simulink model "System3"  (R2025a)
settings: Solver=ode113  StartTime=0.0  StopTime=400  FixedStep=0.01  MaxStep=0.1  RelTol=1e-3
libraries: simulink x3784, slpidlib x2
(part 146 of 160)

== system System3/Battery1/Module3/SubModule_1/Cell14/SOCEstimator/SOCEstimator ==
  SOC_Initial : Inport
  Current : Inport  Port=2
  CellCapacity : Inport  Port=3
  Add1 : Sum  Inputs=+-
  Constant : Constant  Value=100  SampleTime=-1
  Constant1 : Constant  Value=3600  SampleTime=-1
  Delay : Delay  DelayLength=1  InitialConditionSource=Input port
      settings: InputPortMap=u0,p4
  Divide : Product  Inputs=*//
  Divide1 : Product  Inputs=*/
  Integrator : Integrator
  Saturation1 : Saturate  UpperLimit=1  LowerLimit=0
  SOC : Outport
  wires:
  Add1/1 -> Saturation1/1
  Constant/1 -> Divide1/2
  Divide1/1 -> Delay/2, Add1/1
  Divide/1 -> Add1/2
  Saturation1/1 -> Delay/1
  SOC_Initial/1 -> Divide1/1
  Current/1 -> Integrator/1
  Delay/1 -> SOC/1
  CellCapacity/1 -> Divide/2
  Constant1/1 -> Divide/3
  Integrator/1 -> Divide/1

== system System3/Battery1/Module3/SubModule_1/Cell15/2RC/RC1 ==
  Current : Inport
  R : Inport  Port=2
  C : Inport  Port=3
  2 : Constant
  Add : Sum
  Divide : Product  Inputs=*/
  Divide1 : Product  Inputs=*/
  Divide2 : Product  Inputs=/*
  Divide3 : Product  Inputs=**
  Integrator1 : Integrator
  Integrator2 : Integrator
  V : Outport
  wires:
  C/1 -> Divide2/1, Divide1/2
  Integrator1/1 -> Divide/1
  Divide1/1 -> Integrator1/1
  Add/1 -> Divide/2
  R/1 -> Add/1, Divide1/1
  Divide2/1 -> Integrator2/1
  Divide/1 -> Divide3/2
  Current/1 -> Divide3/1
  Divide3/1 -> V/1
  Integrator2/1 -> Add/2
  2/1 -> Divide2/2

== system System3/Battery1/Module3/SubModule_1/Cell15/2RC/RC2 ==
  Current : Inport
  R : Inport  Port=2
  C : Inport  Port=3
  2 : Constant
  Add : Sum
  Divide : Product  Inputs=*/
  Divide1 : Product  Inputs=*/
  Divide2 : Product  Inputs=/*
  Divide3 : Product  Inputs=**
  Integrator1 : Integrator
  Integrator2 : Integrator
  V : Outport
  wires:
  2/1 -> Divide2/2
  Integrator2/1 -> Add/2
  Divide3/1 -> V/1
  Current/1 -> Divide3/1
  Divide/1 -> Divide3/2
  Divide2/1 -> Integrator2/1
  R/1 -> Divide1/1, Add/1
  Add/1 -> Divide/2
  Divide1/1 -> Integrator1/1
  Integrator1/1 -> Divide/1
  C/1 -> Divide1/2, Divide2/1

== system System3/Battery1/Module3/SubModule_1/Cell15/2RC/Rint ==
  Current : Inport
  R : Inport  Port=2
  Divide3 : Product  Inputs=**
  V : Outport
  wires:
  R/1 -> Divide3/2
  Current/1 -> Divide3/1
  Divide3/1 -> V/1

== system System3/Battery1/Module3/SubModule_1/Cell15/SOCEstimator/SOCEstimator ==
  SOC_Initial : Inport
  Current : Inport  Port=2
  CellCapacity : Inport  Port=3
  Add1 : Sum  Inputs=+-
  Constant : Constant  Value=100  SampleTime=-1
  Constant1 : Constant  Value=3600  SampleTime=-1
  Delay : Delay  DelayLength=1  InitialConditionSource=Input port
      settings: InputPortMap=u0,p4
  Divide : Product  Inputs=*//
  Divide1 : Product  Inputs=*/
  Integrator : Integrator
  Saturation1 : Saturate  UpperLimit=1  LowerLimit=0
  SOC : Outport
  wires:
  Add1/1 -> Saturation1/1
  Constant/1 -> Divide1/2
  Divide1/1 -> Delay/2, Add1/1
  Divide/1 -> Add1/2
  Saturation1/1 -> Delay/1
  SOC_Initial/1 -> Divide1/1
  Current/1 -> Integrator/1
  Delay/1 -> SOC/1
  CellCapacity/1 -> Divide/2
  Constant1/1 -> Divide/3
  Integrator/1 -> Divide/1

== system System3/Battery1/Module3/SubModule_1/Cell16/2RC/RC1 ==
  Current : Inport
  R : Inport  Port=2
  C : Inport  Port=3
  2 : Constant
  Add : Sum
  Divide : Product  Inputs=*/
  Divide1 : Product  Inputs=*/
  Divide2 : Product  Inputs=/*
  Divide3 : Product  Inputs=**
  Integrator1 : Integrator
  Integrator2 : Integrator
  V : Outport
  wires:
  C/1 -> Divide2/1, Divide1/2
  Integrator1/1 -> Divide/1
  Divide1/1 -> Integrator1/1
  Add/1 -> Divide/2
  R/1 -> Add/1, Divide1/1
  Divide2/1 -> Integrator2/1
  Divide/1 -> Divide3/2
  Current/1 -> Divide3/1
  Divide3/1 -> V/1
  Integrator2/1 -> Add/2
  2/1 -> Divide2/2

== system System3/Battery1/Module3/SubModule_1/Cell16/2RC/RC2 ==
  Current : Inport
  R : Inport  Port=2
  C : Inport  Port=3
  2 : Constant
  Add : Sum
  Divide : Product  Inputs=*/
  Divide1 : Product  Inputs=*/
  Divide2 : Product  Inputs=/*
  Divide3 : Product  Inputs=**
  Integrator1 : Integrator
  Integrator2 : Integrator
  V : Outport
  wires:
  2/1 -> Divide2/2
  Integrator2/1 -> Add/2
  Divide3/1 -> V/1
  Current/1 -> Divide3/1
  Divide/1 -> Divide3/2
  Divide2/1 -> Integrator2/1
  R/1 -> Divide1/1, Add/1
  Add/1 -> Divide/2
  Divide1/1 -> Integrator1/1
  Integrator1/1 -> Divide/1
  C/1 -> Divide1/2, Divide2/1

== system System3/Battery1/Module3/SubModule_1/Cell16/2RC/Rint ==
  Current : Inport
  R : Inport  Port=2
  Divide3 : Product  Inputs=**
  V : Outport
  wires:
  R/1 -> Divide3/2
  Current/1 -> Divide3/1
  Divide3/1 -> V/1

== system System3/Battery1/Module3/SubModule_1/Cell16/SOCEstimator/SOCEstimator ==
  SOC_Initial : Inport
  Current : Inport  Port=2
  CellCapacity : Inport  Port=3
  Add1 : Sum  Inputs=+-
  Constant : Constant  Value=100  SampleTime=-1
  Constant1 : Constant  Value=3600  SampleTime=-1
  Delay : Delay  DelayLength=1  InitialConditionSource=Input port
      settings: InputPortMap=u0,p4
  Divide : Product  Inputs=*//
  Divide1 : Product  Inputs=*/
  Integrator : Integrator
  Saturation1 : Saturate  UpperLimit=1  LowerLimit=0
  SOC : Outport
  wires:
  Add1/1 -> Saturation1/1
  Constant/1 -> Divide1/2
  Divide1/1 -> Delay/2, Add1/1
  Divide/1 -> Add1/2
  Saturation1/1 -> Delay/1
  SOC_Initial/1 -> Divide1/1
  Current/1 -> Integrator/1
  Delay/1 -> SOC/1
  CellCapacity/1 -> Divide/2
  Constant1/1 -> Divide/3
  Integrator/1 -> Divide/1

== system System3/Battery1/Module3/SubModule_1/Cell17/2RC/RC1 ==
  Current : Inport
  R : Inport  Port=2
  C : Inport  Port=3
  2 : Constant
  Add : Sum
  Divide : Product  Inputs=*/
  Divide1 : Product  Inputs=*/
  Divide2 : Product  Inputs=/*
  Divide3 : Product  Inputs=**
  Integrator1 : Integrator
  Integrator2 : Integrator
  V : Outport
  wires:
  2/1 -> Divide2/2
  Integrator2/1 -> Add/2
  Divide3/1 -> V/1
  Current/1 -> Divide3/1
  Divide/1 -> Divide3/2
  Divide2/1 -> Integrator2/1
  R/1 -> Divide1/1, Add/1
  Add/1 -> Divide/2
  Divide1/1 -> Integrator1/1
  Integrator1/1 -> Divide/1
  C/1 -> Divide1/2, Divide2/1

== system System3/Battery1/Module3/SubModule_1/Cell17/2RC/RC2 ==
  Current : Inport
  R : Inport  Port=2
  C : Inport  Port=3
  2 : Constant
  Add : Sum
  Divide : Product  Inputs=*/
  Divide1 : Product  Inputs=*/
  Divide2 : Product  Inputs=/*
  Divide3 : Product  Inputs=**
  Integrator1 : Integrator
  Integrator2 : Integrator
  V : Outport
  wires:
  C/1 -> Divide2/1, Divide1/2
  Integrator1/1 -> Divide/1
  Divide1/1 -> Integrator1/1
  Add/1 -> Divide/2
  R/1 -> Add/1, Divide1/1
  Divide2/1 -> Integrator2/1
  Divide/1 -> Divide3/2
  Current/1 -> Divide3/1
  Divide3/1 -> V/1
  Integrator2/1 -> Add/2
  2/1 -> Divide2/2

== system System3/Battery1/Module3/SubModule_1/Cell17/2RC/Rint ==
  Current : Inport
  R : Inport  Port=2
  Divide3 : Product  Inputs=**
  V : Outport
  wires:
  Divide3/1 -> V/1
  Current/1 -> Divide3/1
  R/1 -> Divide3/2

== system System3/Battery1/Module3/SubModule_1/Cell17/SOCEstimator/SOCEstimator ==
  SOC_Initial : Inport
  Current : Inport  Port=2
  CellCapacity : Inport  Port=3
  Add1 : Sum  Inputs=+-
  Constant : Constant  Value=100  SampleTime=-1
  Constant1 : Constant  Value=3600  SampleTime=-1
  Delay : Delay  DelayLength=1  InitialConditionSource=Input port
      settings: InputPortMap=u0,p4
  Divide : Product  Inputs=*//
  Divide1 : Product  Inputs=*/
  Integrator : Integrator
  Saturation1 : Saturate  UpperLimit=1  LowerLimit=0
  SOC : Outport
  wires:
  Integrator/1 -> Divide/1
  Constant1/1 -> Divide/3
  CellCapacity/1 -> Divide/2
  Delay/1 -> SOC/1
  Current/1 -> Integrator/1
  SOC_Initial/1 -> Divide1/1
  Saturation1/1 -> Delay/1
  Divide/1 -> Add1/2
  Divide1/1 -> Add1/1, Delay/2
  Constant/1 -> Divide1/2
  Add1/1 -> Saturation1/1

== system System3/Battery1/Module3/SubModule_1/Cell18/2RC/RC1 ==
  Current : Inport
  R : Inport  Port=2
  C : Inport  Port=3
  2 : Constant
  Add : Sum
  Divide : Product  Inputs=*/
  Divide1 : Product  Inputs=*/
  Divide2 : Product  Inputs=/*
  Divide3 : Product  Inputs=**
  Integrator1 : Integrator
  Integrator2 : Integrator
  V : Outport
  wires:
  C/1 -> Divide2/1, Divide1/2
  Integrator1/1 -> Divide/1
  Divide1/1 -> Integrator1/1
  Add/1 -> Divide/2
  R/1 -> Add/1, Divide1/1
  Divide2/1 -> Integrator2/1
  Divide/1 -> Divide3/2
  Current/1 -> Divide3/1
  Divide3/1 -> V/1
  Integrator2/1 -> Add/2
  2/1 -> Divide2/2

== system System3/Battery1/Module3/SubModule_1/Cell18/2RC/RC2 ==
  Current : Inport
  R : Inport  Port=2
  C : Inport  Port=3
  2 : Constant
  Add : Sum
  Divide : Product  Inputs=*/
  Divide1 : Product  Inputs=*/
  Divide2 : Product  Inputs=/*
  Divide3 : Product  Inputs=**
  Integrator1 : Integrator
  Integrator2 : Integrator
  V : Outport
  wires:
  2/1 -> Divide2/2
  Integrator2/1 -> Add/2
  Divide3/1 -> V/1
  Current/1 -> Divide3/1
  Divide/1 -> Divide3/2
  Divide2/1 -> Integrator2/1
  R/1 -> Divide1/1, Add/1
  Add/1 -> Divide/2
  Divide1/1 -> Integrator1/1
  Integrator1/1 -> Divide/1
  C/1 -> Divide1/2, Divide2/1

== system System3/Battery1/Module3/SubModule_1/Cell18/2RC/Rint ==
  Current : Inport
  R : Inport  Port=2
  Divide3 : Product  Inputs=**
  V : Outport
  wires:
  R/1 -> Divide3/2
  Current/1 -> Divide3/1
  Divide3/1 -> V/1

== system System3/Battery1/Module3/SubModule_1/Cell18/SOCEstimator/SOCEstimator ==
  SOC_Initial : Inport
  Current : Inport  Port=2
  CellCapacity : Inport  Port=3
  Add1 : Sum  Inputs=+-
  Constant : Constant  Value=100  SampleTime=-1
  Constant1 : Constant  Value=3600  SampleTime=-1
  Delay : Delay  DelayLength=1  InitialConditionSource=Input port
      settings: InputPortMap=u0,p4
  Divide : Product  Inputs=*//
  Divide1 : Product  Inputs=*/
  Integrator : Integrator
  Saturation1 : Saturate  UpperLimit=1  LowerLimit=0
  SOC : Outport
  wires:
  Add1/1 -> Saturation1/1
  Constant/1 -> Divide1/2
  Divide1/1 -> Delay/2, Add1/1
  Divide/1 -> Add1/2
  Saturation1/1 -> Delay/1
  SOC_Initial/1 -> Divide1/1
  Current/1 -> Integrator/1
  Delay/1 -> SOC/1
  CellCapacity/1 -> Divide/2
  Constant1/1 -> Divide/3
  Integrator/1 -> Divide/1

== system System3/Battery1/Module3/SubModule_1/Cell19/2RC/RC1 ==
  Current : Inport
  R : Inport  Port=2
  C : Inport  Port=3
  2 : Constant
  Add : Sum
  Divide : Product  Inputs=*/
  Divide1 : Product  Inputs=*/
  Divide2 : Product  Inputs=/*
  Divide3 : Product  Inputs=**
  Integrator1 : Integrator
  Integrator2 : Integrator
  V : Outport
  wires:
  2/1 -> Divide2/2
  Integrator2/1 -> Add/2
  Divide3/1 -> V/1
  Current/1 -> Divide3/1
  Divide/1 -> Divide3/2
  Divide2/1 -> Integrator2/1
  R/1 -> Divide1/1, Add/1
  Add/1 -> Divide/2
  Divide1/1 -> Integrator1/1
  Integrator1/1 -> Divide/1
  C/1 -> Divide1/2, Divide2/1

== system System3/Battery1/Module3/SubModule_1/Cell19/2RC/RC2 ==
  Current : Inport
  R : Inport  Port=2
  C : Inport  Port=3
  2 : Constant
  Add : Sum
  Divide : Product  Inputs=*/
  Divide1 : Product  Inputs=*/
  Divide2 : Product  Inputs=/*
  Divide3 : Product  Inputs=**
  Integrator1 : Integrator
  Integrator2 : Integrator
  V : Outport
  wires:
  C/1 -> Divide2/1, Divide1/2
  Integrator1/1 -> Divide/1
  Divide1/1 -> Integrator1/1
  Add/1 -> Divide/2
  R/1 -> Add/1, Divide1/1
  Divide2/1 -> Integrator2/1
  Divide/1 -> Divide3/2
  Current/1 -> Divide3/1
  Divide3/1 -> V/1
  Integrator2/1 -> Add/2
  2/1 -> Divide2/2

== system System3/Battery1/Module3/SubModule_1/Cell19/2RC/Rint ==
  Current : Inport
  R : Inport  Port=2
  Divide3 : Product  Inputs=**
  V : Outport
  wires:
  Divide3/1 -> V/1
  Current/1 -> Divide3/1
  R/1 -> Divide3/2

== system System3/Battery1/Module3/SubModule_1/Cell19/SOCEstimator/SOCEstimator ==
  SOC_Initial : Inport
  Current : Inport  Port=2
  CellCapacity : Inport  Port=3
  Add1 : Sum  Inputs=+-
  Constant : Constant  Value=100  SampleTime=-1
  Constant1 : Constant  Value=3600  SampleTime=-1
  Delay : Delay  DelayLength=1  InitialConditionSource=Input port
      settings: InputPortMap=u0,p4
  Divide : Product  Inputs=*//
  Divide1 : Product  Inputs=*/
  Integrator : Integrator
  Saturation1 : Saturate  UpperLimit=1  LowerLimit=0
  SOC : Outport
  wires:
  Integrator/1 -> Divide/1
  Constant1/1 -> Divide/3
  CellCapacity/1 -> Divide/2
  Delay/1 -> SOC/1
  Current/1 -> Integrator/1
  SOC_Initial/1 -> Divide1/1
  Saturation1/1 -> Delay/1
  Divide/1 -> Add1/2
  Divide1/1 -> Add1/1, Delay/2
  Constant/1 -> Divide1/2
  Add1/1 -> Saturation1/1

== system System3/Battery1/Module3/SubModule_1/Cell2/2RC/RC1 ==
  Current : Inport
  R : Inport  Port=2
  C : Inport  Port=3
  2 : Constant
  Add : Sum
  Divide : Product  Inputs=*/
  Divide1 : Product  Inputs=*/
  Divide2 : Product  Inputs=/*
  Divide3 : Product  Inputs=**
  Integrator1 : Integrator
  Integrator2 : Integrator
  V : Outport
  wires:
  C/1 -> Divide2/1, Divide1/2
  Integrator1/1 -> Divide/1
  Divide1/1 -> Integrator1/1
  Add/1 -> Divide/2
  R/1 -> Add/1, Divide1/1
  Divide2/1 -> Integrator2/1
  Divide/1 -> Divide3/2
  Current/1 -> Divide3/1
  Divide3/1 -> V/1
  Integrator2/1 -> Add/2
  2/1 -> Divide2/2

== system System3/Battery1/Module3/SubModule_1/Cell2/2RC/RC2 ==
  Current : Inport
  R : Inport  Port=2
  C : Inport  Port=3
  2 : Constant
  Add : Sum
  Divide : Product  Inputs=*/
  Divide1 : Product  Inputs=*/
  Divide2 : Product  Inputs=/*
  Divide3 : Product  Inputs=**
  Integrator1 : Integrator
  Integrator2 : Integrator
  V : Outport
  wires:
  2/1 -> Divide2/2
  Integrator2/1 -> Add/2
  Divide3/1 -> V/1
  Current/1 -> Divide3/1
  Divide/1 -> Divide3/2
  Divide2/1 -> Integrator2/1
  R/1 -> Divide1/1, Add/1
  Add/1 -> Divide/2
  Divide1/1 -> Integrator1/1
  Integrator1/1 -> Divide/1
  C/1 -> Divide1/2, Divide2/1

== system System3/Battery1/Module3/SubModule_1/Cell2/2RC/Rint ==
  Current : Inport
  R : Inport  Port=2
  Divide3 : Product  Inputs=**
  V : Outport
  wires:
  R/1 -> Divide3/2
  Current/1 -> Divide3/1
  Divide3/1 -> V/1

== system System3/Battery1/Module3/SubModule_1/Cell2/SOCEstimator/SOCEstimator ==
  SOC_Initial : Inport
  Current : Inport  Port=2
  CellCapacity : Inport  Port=3
  Add1 : Sum  Inputs=+-
  Constant : Constant  Value=100  SampleTime=-1
  Constant1 : Constant  Value=3600  SampleTime=-1
  Delay : Delay  DelayLength=1  InitialConditionSource=Input port
      settings: InputPortMap=u0,p4
  Divide : Product  Inputs=*//
  Divide1 : Product  Inputs=*/
  Integrator : Integrator
  Saturation1 : Saturate  UpperLimit=1  LowerLimit=0
  SOC : Outport
  wires:
  Add1/1 -> Saturation1/1
  Constant/1 -> Divide1/2
  Divide1/1 -> Delay/2, Add1/1
  Divide/1 -> Add1/2
  Saturation1/1 -> Delay/1
  SOC_Initial/1 -> Divide1/1
  Current/1 -> Integrator/1
  Delay/1 -> SOC/1
  CellCapacity/1 -> Divide/2
  Constant1/1 -> Divide/3
  Integrator/1 -> Divide/1

== system System3/Battery1/Module3/SubModule_1/Cell20/2RC/RC1 ==
  Current : Inport
  R : Inport  Port=2
  C : Inport  Port=3
  2 : Constant
  Add : Sum
  Divide : Product  Inputs=*/
  Divide1 : Product  Inputs=*/
  Divide2 : Product  Inputs=/*
  Divide3 : Product  Inputs=**
  Integrator1 : Integrator
  Integrator2 : Integrator
  V : Outport
  wires:
  C/1 -> Divide2/1, Divide1/2
  Integrator1/1 -> Divide/1
  Divide1/1 -> Integrator1/1
  Add/1 -> Divide/2
  R/1 -> Add/1, Divide1/1
  Divide2/1 -> Integrator2/1
  Divide/1 -> Divide3/2
  Current/1 -> Divide3/1
  Divide3/1 -> V/1
  Integrator2/1 -> Add/2
  2/1 -> Divide2/2

== system System3/Battery1/Module3/SubModule_1/Cell20/2RC/RC2 ==
  Current : Inport
  R : Inport  Port=2
  C : Inport  Port=3
  2 : Constant
  Add : Sum
  Divide : Product  Inputs=*/
  Divide1 : Product  Inputs=*/
  Divide2 : Product  Inputs=/*
  Divide3 : Product  Inputs=**
  Integrator1 : Integrator
  Integrator2 : Integrator
  V : Outport
  wires:
  2/1 -> Divide2/2
  Integrator2/1 -> Add/2
  Divide3/1 -> V/1
  Current/1 -> Divide3/1
  Divide/1 -> Divide3/2
  Divide2/1 -> Integrator2/1
  R/1 -> Divide1/1, Add/1
  Add/1 -> Divide/2
  Divide1/1 -> Integrator1/1
  Integrator1/1 -> Divide/1
  C/1 -> Divide1/2, Divide2/1

== system System3/Battery1/Module3/SubModule_1/Cell20/2RC/Rint ==
  Current : Inport
  R : Inport  Port=2
  Divide3 : Product  Inputs=**
  V : Outport
  wires:
  R/1 -> Divide3/2
  Current/1 -> Divide3/1
  Divide3/1 -> V/1

== system System3/Battery1/Module3/SubModule_1/Cell20/SOCEstimator/SOCEstimator ==
  SOC_Initial : Inport
  Current : Inport  Port=2
  CellCapacity : Inport  Port=3
  Add1 : Sum  Inputs=+-
  Constant : Constant  Value=100  SampleTime=-1
  Constant1 : Constant  Value=3600  SampleTime=-1
  Delay : Delay  DelayLength=1  InitialConditionSource=Input port
      settings: InputPortMap=u0,p4
  Divide : Product  Inputs=*//
  Divide1 : Product  Inputs=*/
  Integrator : Integrator
  Saturation1 : Saturate  UpperLimit=1  LowerLimit=0
  SOC : Outport
  wires:
  Add1/1 -> Saturation1/1
  Constant/1 -> Divide1/2
  Divide1/1 -> Delay/2, Add1/1
  Divide/1 -> Add1/2
  Saturation1/1 -> Delay/1
  SOC_Initial/1 -> Divide1/1
  Current/1 -> Integrator/1
  Delay/1 -> SOC/1
  CellCapacity/1 -> Divide/2
  Constant1/1 -> Divide/3
  Integrator/1 -> Divide/1

== system System3/Battery1/Module3/SubModule_1/Cell21/2RC/RC1 ==
  Current : Inport
  R : Inport  Port=2
  C : Inport  Port=3
  2 : Constant
  Add : Sum
  Divide : Product  Inputs=*/
  Divide1 : Product  Inputs=*/
  Divide2 : Product  Inputs=/*
  Divide3 : Product  Inputs=**
  Integrator1 : Integrator
  Integrator2 : Integrator
  V : Outport
  wires:
  2/1 -> Divide2/2
  Integrator2/1 -> Add/2
  Divide3/1 -> V/1
  Current/1 -> Divide3/1
  Divide/1 -> Divide3/2
  Divide2/1 -> Integrator2/1
  R/1 -> Divide1/1, Add/1
  Add/1 -> Divide/2
  Divide1/1 -> Integrator1/1
  Integrator1/1 -> Divide/1
  C/1 -> Divide1/2, Divide2/1

== system System3/Battery1/Module3/SubModule_1/Cell21/2RC/RC2 ==
  Current : Inport
  R : Inport  Port=2
  C : Inport  Port=3
  2 : Constant
  Add : Sum
  Divide : Product  Inputs=*/
  Divide1 : Product  Inputs=*/
  Divide2 : Product  Inputs=/*
  Divide3 : Product  Inputs=**
  Integrator1 : Integrator
  Integrator2 : Integrator
  V : Outport
  wires:
  C/1 -> Divide2/1, Divide1/2
  Integrator1/1 -> Divide/1
  Divide1/1 -> Integrator1/1
  Add/1 -> Divide/2
  R/1 -> Add/1, Divide1/1
  Divide2/1 -> Integrator2/1
  Divide/1 -> Divide3/2
  Current/1 -> Divide3/1
  Divide3/1 -> V/1
  Integrator2/1 -> Add/2
  2/1 -> Divide2/2

== system System3/Battery1/Module3/SubModule_1/Cell21/2RC/Rint ==
  Current : Inport
  R : Inport  Port=2
  Divide3 : Product  Inputs=**
  V : Outport
  wires:
  Divide3/1 -> V/1
  Current/1 -> Divide3/1
  R/1 -> Divide3/2

== system System3/Battery1/Module3/SubModule_1/Cell21/SOCEstimator/SOCEstimator ==
  SOC_Initial : Inport
  Current : Inport  Port=2
  CellCapacity : Inport  Port=3
  Add1 : Sum  Inputs=+-
  Constant : Constant  Value=100  SampleTime=-1
  Constant1 : Constant  Value=3600  SampleTime=-1
  Delay : Delay  DelayLength=1  InitialConditionSource=Input port
      settings: InputPortMap=u0,p4
  Divide : Product  Inputs=*//
  Divide1 : Product  Inputs=*/
  Integrator : Integrator
  Saturation1 : Saturate  UpperLimit=1  LowerLimit=0
  SOC : Outport
  wires:
  Integrator/1 -> Divide/1
  Constant1/1 -> Divide/3
  CellCapacity/1 -> Divide/2
  Delay/1 -> SOC/1
  Current/1 -> Integrator/1
  SOC_Initial/1 -> Divide1/1
  Saturation1/1 -> Delay/1
  Divide/1 -> Add1/2
  Divide1/1 -> Add1/1, Delay/2
  Constant/1 -> Divide1/2
  Add1/1 -> Saturation1/1

== system System3/Battery1/Module3/SubModule_1/Cell22/2RC/RC1 ==
  Current : Inport
  R : Inport  Port=2
  C : Inport  Port=3
  2 : Constant
  Add : Sum
  Divide : Product  Inputs=*/
  Divide1 : Product  Inputs=*/
  Divide2 : Product  Inputs=/*
  Divide3 : Product  Inputs=**
  Integrator1 : Integrator
  Integrator2 : Integrator
  V : Outport
  wires:
  2/1 -> Divide2/2
  Integrator2/1 -> Add/2
  Divide3/1 -> V/1
  Current/1 -> Divide3/1
  Divide/1 -> Divide3/2
  Divide2/1 -> Integrator2/1
  R/1 -> Divide1/1, Add/1
  Add/1 -> Divide/2
  Divide1/1 -> Integrator1/1
  Integrator1/1 -> Divide/1
  C/1 -> Divide1/2, Divide2/1

== system System3/Battery1/Module3/SubModule_1/Cell22/2RC/RC2 ==
  Current : Inport
  R : Inport  Port=2
  C : Inport  Port=3
  2 : Constant
  Add : Sum
  Divide : Product  Inputs=*/
  Divide1 : Product  Inputs=*/
  Divide2 : Product  Inputs=/*
  Divide3 : Product  Inputs=**
  Integrator1 : Integrator
  Integrator2 : Integrator
  V : Outport
  wires:
  C/1 -> Divide2/1, Divide1/2
  Integrator1/1 -> Divide/1
  Divide1/1 -> Integrator1/1
  Add/1 -> Divide/2
  R/1 -> Add/1, Divide1/1
  Divide2/1 -> Integrator2/1
  Divide/1 -> Divide3/2
  Current/1 -> Divide3/1
  Divide3/1 -> V/1
  Integrator2/1 -> Add/2
  2/1 -> Divide2/2

== system System3/Battery1/Module3/SubModule_1/Cell22/2RC/Rint ==
  Current : Inport
  R : Inport  Port=2
  Divide3 : Product  Inputs=**
  V : Outport
  wires:
  Divide3/1 -> V/1
  Current/1 -> Divide3/1
  R/1 -> Divide3/2

== system System3/Battery1/Module3/SubModule_1/Cell22/SOCEstimator/SOCEstimator ==
  SOC_Initial : Inport
  Current : Inport  Port=2
  CellCapacity : Inport  Port=3
  Add1 : Sum  Inputs=+-
  Constant : Constant  Value=100  SampleTime=-1
  Constant1 : Constant  Value=3600  SampleTime=-1
  Delay : Delay  DelayLength=1  InitialConditionSource=Input port
      settings: InputPortMap=u0,p4
  Divide : Product  Inputs=*//
  Divide1 : Product  Inputs=*/
  Integrator : Integrator
  Saturation1 : Saturate  UpperLimit=1  LowerLimit=0
  SOC : Outport
  wires:
  Integrator/1 -> Divide/1
  Constant1/1 -> Divide/3
  CellCapacity/1 -> Divide/2
  Delay/1 -> SOC/1
  Current/1 -> Integrator/1
  SOC_Initial/1 -> Divide1/1
  Saturation1/1 -> Delay/1
  Divide/1 -> Add1/2
  Divide1/1 -> Add1/1, Delay/2
  Constant/1 -> Divide1/2
  Add1/1 -> Saturation1/1

== system System3/Battery1/Module3/SubModule_1/Cell3/2RC/RC1 ==
  Current : Inport
  R : Inport  Port=2
  C : Inport  Port=3
  2 : Constant
  Add : Sum
  Divide : Product  Inputs=*/
  Divide1 : Product  Inputs=*/
  Divide2 : Product  Inputs=/*
  Divide3 : Product  Inputs=**
  Integrator1 : Integrator
  Integrator2 : Integrator
  V : Outport
  wires:
  2/1 -> Divide2/2
  Integrator2/1 -> Add/2
  Divide3/1 -> V/1
  Current/1 -> Divide3/1
  Divide/1 -> Divide3/2
  Divide2/1 -> Integrator2/1
  R/1 -> Divide1/1, Add/1
  Add/1 -> Divide/2
  Divide1/1 -> Integrator1/1
  Integrator1/1 -> Divide/1
  C/1 -> Divide1/2, Divide2/1

== system System3/Battery1/Module3/SubModule_1/Cell3/2RC/RC2 ==
  Current : Inport
  R : Inport  Port=2
  C : Inport  Port=3
  2 : Constant
  Add : Sum
  Divide : Product  Inputs=*/
  Divide1 : Product  Inputs=*/
  Divide2 : Product  Inputs=/*
  Divide3 : Product  Inputs=**
  Integrator1 : Integrator
  Integrator2 : Integrator
  V : Outport
  wires:
  C/1 -> Divide2/1, Divide1/2
  Integrator1/1 -> Divide/1
  Divide1/1 -> Integrator1/1
  Add/1 -> Divide/2
  R/1 -> Add/1, Divide1/1
  Divide2/1 -> Integrator2/1
  Divide/1 -> Divide3/2
  Current/1 -> Divide3/1
  Divide3/1 -> V/1
  Integrator2/1 -> Add/2
  2/1 -> Divide2/2

== system System3/Battery1/Module3/SubModule_1/Cell3/2RC/Rint ==
  Current : Inport
  R : Inport  Port=2
  Divide3 : Product  Inputs=**
  V : Outport
  wires:
  Divide3/1 -> V/1
  Current/1 -> Divide3/1
  R/1 -> Divide3/2

== system System3/Battery1/Module3/SubModule_1/Cell3/SOCEstimator/SOCEstimator ==
  SOC_Initial : Inport
  Current : Inport  Port=2
  CellCapacity : Inport  Port=3
  Add1 : Sum  Inputs=+-
  Constant : Constant  Value=100  SampleTime=-1
  Constant1 : Constant  Value=3600  SampleTime=-1
  Delay : Delay  DelayLength=1  InitialConditionSource=Input port
      settings: InputPortMap=u0,p4
  Divide : Product  Inputs=*//
  Divide1 : Product  Inputs=*/
  Integrator : Integrator
  Saturation1 : Saturate  UpperLimit=1  LowerLimit=0
  SOC : Outport
  wires:
  Integrator/1 -> Divide/1
  Constant1/1 -> Divide/3
  CellCapacity/1 -> Divide/2
  Delay/1 -> SOC/1
  Current/1 -> Integrator/1
  SOC_Initial/1 -> Divide1/1
  Saturation1/1 -> Delay/1
  Divide/1 -> Add1/2
  Divide1/1 -> Add1/1, Delay/2
  Constant/1 -> Divide1/2
  Add1/1 -> Saturation1/1

== system System3/Battery1/Module3/SubModule_1/Cell4/2RC/RC1 ==
  Current : Inport
  R : Inport  Port=2
  C : Inport  Port=3
  2 : Constant
  Add : Sum
  Divide : Product  Inputs=*/
  Divide1 : Product  Inputs=*/
  Divide2 : Product  Inputs=/*
  Divide3 : Product  Inputs=**
  Integrator1 : Integrator
  Integrator2 : Integrator
  V : Outport
  wires:
  C/1 -> Divide2/1, Divide1/2
  Integrator1/1 -> Divide/1
  Divide1/1 -> Integrator1/1
  Add/1 -> Divide/2
  R/1 -> Add/1, Divide1/1
  Divide2/1 -> Integrator2/1
  Divide/1 -> Divide3/2
  Current/1 -> Divide3/1
  Divide3/1 -> V/1
  Integrator2/1 -> Add/2
  2/1 -> Divide2/2

== system System3/Battery1/Module3/SubModule_1/Cell4/2RC/RC2 ==
  Current : Inport
  R : Inport  Port=2
  C : Inport  Port=3
  2 : Constant
  Add : Sum
  Divide : Product  Inputs=*/
  Divide1 : Product  Inputs=*/
  Divide2 : Product  Inputs=/*
  Divide3 : Product  Inputs=**
  Integrator1 : Integrator
  Integrator2 : Integrator
  V : Outport
  wires:
  2/1 -> Divide2/2
  Integrator2/1 -> Add/2
  Divide3/1 -> V/1
  Current/1 -> Divide3/1
  Divide/1 -> Divide3/2
  Divide2/1 -> Integrator2/1
  R/1 -> Divide1/1, Add/1
  Add/1 -> Divide/2
  Divide1/1 -> Integrator1/1
  Integrator1/1 -> Divide/1
  C/1 -> Divide1/2, Divide2/1

== system System3/Battery1/Module3/SubModule_1/Cell4/2RC/Rint ==
  Current : Inport
  R : Inport  Port=2
  Divide3 : Product  Inputs=**
  V : Outport
  wires:
  R/1 -> Divide3/2
  Current/1 -> Divide3/1
  Divide3/1 -> V/1

== system System3/Battery1/Module3/SubModule_1/Cell4/SOCEstimator/SOCEstimator ==
  SOC_Initial : Inport
  Current : Inport  Port=2
  CellCapacity : Inport  Port=3
  Add1 : Sum  Inputs=+-
  Constant : Constant  Value=100  SampleTime=-1
  Constant1 : Constant  Value=3600  SampleTime=-1
  Delay : Delay  DelayLength=1  InitialConditionSource=Input port
      settings: InputPortMap=u0,p4
  Divide : Product  Inputs=*//
  Divide1 : Product  Inputs=*/
  Integrator : Integrator
  Saturation1 : Saturate  UpperLimit=1  LowerLimit=0
  SOC : Outport
  wires:
  Add1/1 -> Saturation1/1
  Constant/1 -> Divide1/2
  Divide1/1 -> Delay/2, Add1/1
  Divide/1 -> Add1/2
  Saturation1/1 -> Delay/1
  SOC_Initial/1 -> Divide1/1
  Current/1 -> Integrator/1
  Delay/1 -> SOC/1
  CellCapacity/1 -> Divide/2
  Constant1/1 -> Divide/3
  Integrator/1 -> Divide/1

== system System3/Battery1/Module3/SubModule_1/Cell5/2RC/RC1 ==
  Current : Inport
  R : Inport  Port=2
  C : Inport  Port=3
  2 : Constant
  Add : Sum
  Divide : Product  Inputs=*/
  Divide1 : Product  Inputs=*/
  Divide2 : Product  Inputs=/*
  Divide3 : Product  Inputs=**
  Integrator1 : Integrator
  Integrator2 : Integrator
  V : Outport
  wires:
  2/1 -> Divide2/2
  Integrator2/1 -> Add/2
  Divide3/1 -> V/1
  Current/1 -> Divide3/1
  Divide/1 -> Divide3/2
  Divide2/1 -> Integrator2/1
  R/1 -> Divide1/1, Add/1
  Add/1 -> Divide/2
  Divide1/1 -> Integrator1/1
  Integrator1/1 -> Divide/1
  C/1 -> Divide1/2, Divide2/1

== system System3/Battery1/Module3/SubModule_1/Cell5/2RC/RC2 ==
  Current : Inport
  R : Inport  Port=2
  C : Inport  Port=3
  2 : Constant
  Add : Sum
  Divide : Product  Inputs=*/
  Divide1 : Product  Inputs=*/
  Divide2 : Product  Inputs=/*
  Divide3 : Product  Inputs=**
  Integrator1 : Integrator
  Integrator2 : Integrator
  V : Outport
  wires:
  C/1 -> Divide2/1, Divide1/2
  Integrator1/1 -> Divide/1
  Divide1/1 -> Integrator1/1
  Add/1 -> Divide/2
  R/1 -> Add/1, Divide1/1
  Divide2/1 -> Integrator2/1
  Divide/1 -> Divide3/2
  Current/1 -> Divide3/1
  Divide3/1 -> V/1
  Integrator2/1 -> Add/2
  2/1 -> Divide2/2

== system System3/Battery1/Module3/SubModule_1/Cell5/2RC/Rint ==
  Current : Inport
  R : Inport  Port=2
  Divide3 : Product  Inputs=**
  V : Outport
  wires:
  Divide3/1 -> V/1
  Current/1 -> Divide3/1
  R/1 -> Divide3/2

== system System3/Battery1/Module3/SubModule_1/Cell5/SOCEstimator/SOCEstimator ==
  SOC_Initial : Inport
  Current : Inport  Port=2
  CellCapacity : Inport  Port=3
  Add1 : Sum  Inputs=+-
  Constant : Constant  Value=100  SampleTime=-1
  Constant1 : Constant  Value=3600  SampleTime=-1
  Delay : Delay  DelayLength=1  InitialConditionSource=Input port
      settings: InputPortMap=u0,p4
  Divide : Product  Inputs=*//
  Divide1 : Product  Inputs=*/
  Integrator : Integrator
  Saturation1 : Saturate  UpperLimit=1  LowerLimit=0
  SOC : Outport
  wires:
  Integrator/1 -> Divide/1
  Constant1/1 -> Divide/3
  CellCapacity/1 -> Divide/2
  Delay/1 -> SOC/1
  Current/1 -> Integrator/1
  SOC_Initial/1 -> Divide1/1
  Saturation1/1 -> Delay/1
  Divide/1 -> Add1/2
  Divide1/1 -> Add1/1, Delay/2
  Constant/1 -> Divide1/2
  Add1/1 -> Saturation1/1

== system System3/Battery1/Module3/SubModule_1/Cell6/2RC/RC1 ==
  Current : Inport
  R : Inport  Port=2
  C : Inport  Port=3
  2 : Constant
  Add : Sum
  Divide : Product  Inputs=*/
  Divide1 : Product  Inputs=*/
  Divide2 : Product  Inputs=/*
  Divide3 : Product  Inputs=**
  Integrator1 : Integrator
  Integrator2 : Integrator
  V : Outport
  wires:
  C/1 -> Divide2/1, Divide1/2
  Integrator1/1 -> Divide/1
  Divide1/1 -> Integrator1/1
  Add/1 -> Divide/2
  R/1 -> Add/1, Divide1/1
  Divide2/1 -> Integrator2/1
  Divide/1 -> Divide3/2
  Current/1 -> Divide3/1
  Divide3/1 -> V/1
  Integrator2/1 -> Add/2
  2/1 -> Divide2/2

== system System3/Battery1/Module3/SubModule_1/Cell6/2RC/RC2 ==
  Current : Inport
  R : Inport  Port=2
  C : Inport  Port=3
  2 : Constant
  Add : Sum
  Divide : Product  Inputs=*/
  Divide1 : Product  Inputs=*/
  Divide2 : Product  Inputs=/*
  Divide3 : Product  Inputs=**
  Integrator1 : Integrator
  Integrator2 : Integrator
  V : Outport
  wires:
  2/1 -> Divide2/2
  Integrator2/1 -> Add/2
  Divide3/1 -> V/1
  Current/1 -> Divide3/1
  Divide/1 -> Divide3/2
  Divide2/1 -> Integrator2/1
  R/1 -> Divide1/1, Add/1
  Add/1 -> Divide/2
  Divide1/1 -> Integrator1/1
  Integrator1/1 -> Divide/1
  C/1 -> Divide1/2, Divide2/1

== system System3/Battery1/Module3/SubModule_1/Cell6/2RC/Rint ==
  Current : Inport
  R : Inport  Port=2
  Divide3 : Product  Inputs=**
  V : Outport
  wires:
  R/1 -> Divide3/2
  Current/1 -> Divide3/1
  Divide3/1 -> V/1

== system System3/Battery1/Module3/SubModule_1/Cell6/SOCEstimator/SOCEstimator ==
  SOC_Initial : Inport
  Current : Inport  Port=2
  CellCapacity : Inport  Port=3
  Add1 : Sum  Inputs=+-
  Constant : Constant  Value=100  SampleTime=-1
  Constant1 : Constant  Value=3600  SampleTime=-1
  Delay : Delay  DelayLength=1  InitialConditionSource=Input port
      settings: InputPortMap=u0,p4
  Divide : Product  Inputs=*//
  Divide1 : Product  Inputs=*/
  Integrator : Integrator
  Saturation1 : Saturate  UpperLimit=1  LowerLimit=0
  SOC : Outport
  wires:
  Add1/1 -> Saturation1/1
  Constant/1 -> Divide1/2
  Divide1/1 -> Delay/2, Add1/1
  Divide/1 -> Add1/2
  Saturation1/1 -> Delay/1
  SOC_Initial/1 -> Divide1/1
  Current/1 -> Integrator/1
  Delay/1 -> SOC/1
  CellCapacity/1 -> Divide/2
  Constant1/1 -> Divide/3
  Integrator/1 -> Divide/1

== system System3/Battery1/Module3/SubModule_1/Cell7/2RC/RC1 ==
  Current : Inport
  R : Inport  Port=2
  C : Inport  Port=3
  2 : Constant
  Add : Sum
  Divide : Product  Inputs=*/
  Divide1 : Product  Inputs=*/
  Divide2 : Product  Inputs=/*
  Divide3 : Product  Inputs=**
  Integrator1 : Integrator
  Integrator2 : Integrator
  V : Outport
  wires:
  C/1 -> Divide2/1, Divide1/2
  Integrator1/1 -> Divide/1
  Divide1/1 -> Integrator1/1
  Add/1 -> Divide/2
  R/1 -> Add/1, Divide1/1
  Divide2/1 -> Integrator2/1
  Divide/1 -> Divide3/2
  Current/1 -> Divide3/1
  Divide3/1 -> V/1
  Integrator2/1 -> Add/2
  2/1 -> Divide2/2

== system System3/Battery1/Module3/SubModule_1/Cell7/2RC/RC2 ==
  Current : Inport
  R : Inport  Port=2
  C : Inport  Port=3
  2 : Constant
  Add : Sum
  Divide : Product  Inputs=*/
  Divide1 : Product  Inputs=*/
  Divide2 : Product  Inputs=/*
  Divide3 : Product  Inputs=**
  Integrator1 : Integrator
  Integrator2 : Integrator
  V : Outport
  wires:
  2/1 -> Divide2/2
  Integrator2/1 -> Add/2
  Divide3/1 -> V/1
  Current/1 -> Divide3/1
  Divide/1 -> Divide3/2
  Divide2/1 -> Integrator2/1
  R/1 -> Divide1/1, Add/1
  Add/1 -> Divide/2
  Divide1/1 -> Integrator1/1
  Integrator1/1 -> Divide/1
  C/1 -> Divide1/2, Divide2/1

== system System3/Battery1/Module3/SubModule_1/Cell7/2RC/Rint ==
  Current : Inport
  R : Inport  Port=2
  Divide3 : Product  Inputs=**
  V : Outport
  wires:
  R/1 -> Divide3/2
  Current/1 -> Divide3/1
  Divide3/1 -> V/1

== system System3/Battery1/Module3/SubModule_1/Cell7/SOCEstimator/SOCEstimator ==
  SOC_Initial : Inport
  Current : Inport  Port=2
  CellCapacity : Inport  Port=3
  Add1 : Sum  Inputs=+-
  Constant : Constant  Value=100  SampleTime=-1
  Constant1 : Constant  Value=3600  SampleTime=-1
  Delay : Delay  DelayLength=1  InitialConditionSource=Input port
      settings: InputPortMap=u0,p4
  Divide : Product  Inputs=*//
  Divide1 : Product  Inputs=*/
  Integrator : Integrator
  Saturation1 : Saturate  UpperLimit=1  LowerLimit=0
  SOC : Outport
  wires:
  Add1/1 -> Saturation1/1
  Constant/1 -> Divide1/2
  Divide1/1 -> Delay/2, Add1/1
  Divide/1 -> Add1/2
  Saturation1/1 -> Delay/1
  SOC_Initial/1 -> Divide1/1
  Current/1 -> Integrator/1
  Delay/1 -> SOC/1
  CellCapacity/1 -> Divide/2
  Constant1/1 -> Divide/3
  Integrator/1 -> Divide/1

== system System3/Battery1/Module3/SubModule_1/Cell8/2RC/RC1 ==
  Current : Inport
  R : Inport  Port=2
  C : Inport  Port=3
  2 : Constant
  Add : Sum
  Divide : Product  Inputs=*/
  Divide1 : Product  Inputs=*/
  Divide2 : Product  Inputs=/*
  Divide3 : Product  Inputs=**
  Integrator1 : Integrator
  Integrator2 : Integrator
  V : Outport
  wires:
  2/1 -> Divide2/2
  Integrator2/1 -> Add/2
  Divide3/1 -> V/1
  Current/1 -> Divide3/1
  Divide/1 -> Divide3/2
  Divide2/1 -> Integrator2/1
  R/1 -> Divide1/1, Add/1
  Add/1 -> Divide/2
  Divide1/1 -> Integrator1/1
  Integrator1/1 -> Divide/1
  C/1 -> Divide1/2, Divide2/1

== system System3/Battery1/Module3/SubModule_1/Cell8/2RC/RC2 ==
  Current : Inport
  R : Inport  Port=2
  C : Inport  Port=3
  2 : Constant
  Add : Sum
  Divide : Product  Inputs=*/
  Divide1 : Product  Inputs=*/
  Divide2 : Product  Inputs=/*
  Divide3 : Product  Inputs=**
  Integrator1 : Integrator
  Integrator2 : Integrator
  V : Outport
  wires:
  C/1 -> Divide2/1, Divide1/2
  Integrator1/1 -> Divide/1
  Divide1/1 -> Integrator1/1
  Add/1 -> Divide/2
  R/1 -> Add/1, Divide1/1
  Divide2/1 -> Integrator2/1
  Divide/1 -> Divide3/2
  Current/1 -> Divide3/1
  Divide3/1 -> V/1
  Integrator2/1 -> Add/2
  2/1 -> Divide2/2

== system System3/Battery1/Module3/SubModule_1/Cell8/2RC/Rint ==
  Current : Inport
  R : Inport  Port=2
  Divide3 : Product  Inputs=**
  V : Outport
  wires:
  Divide3/1 -> V/1
  Current/1 -> Divide3/1
  R/1 -> Divide3/2

== system System3/Battery1/Module3/SubModule_1/Cell8/SOCEstimator/SOCEstimator ==
  SOC_Initial : Inport
  Current : Inport  Port=2
  CellCapacity : Inport  Port=3
  Add1 : Sum  Inputs=+-
  Constant : Constant  Value=100  SampleTime=-1
  Constant1 : Constant  Value=3600  SampleTime=-1
  Delay : Delay  DelayLength=1  InitialConditionSource=Input port
      settings: InputPortMap=u0,p4
  Divide : Product  Inputs=*//
  Divide1 : Product  Inputs=*/
  Integrator : Integrator
  Saturation1 : Saturate  UpperLimit=1  LowerLimit=0
  SOC : Outport
  wires:
  Integrator/1 -> Divide/1
  Constant1/1 -> Divide/3
  CellCapacity/1 -> Divide/2
  Delay/1 -> SOC/1
  Current/1 -> Integrator/1
  SOC_Initial/1 -> Divide1/1
  Saturation1/1 -> Delay/1
  Divide/1 -> Add1/2
  Divide1/1 -> Add1/1, Delay/2
  Constant/1 -> Divide1/2
  Add1/1 -> Saturation1/1

== system System3/Battery1/Module3/SubModule_1/Cell9/2RC/RC1 ==
  Current : Inport
  R : Inport  Port=2
  C : Inport  Port=3
  2 : Constant
  Add : Sum
  Divide : Product  Inputs=*/
  Divide1 : Product  Inputs=*/
  Divide2 : Product  Inputs=/*
  Divide3 : Product  Inputs=**
  Integrator1 : Integrator
  Integrator2 : Integrator
  V : Outport
  wires:
  C/1 -> Divide2/1, Divide1/2
  Integrator1/1 -> Divide/1
  Divide1/1 -> Integrator1/1
  Add/1 -> Divide/2
  R/1 -> Add/1, Divide1/1
  Divide2/1 -> Integrator2/1
  Divide/1 -> Divide3/2
  Current/1 -> Divide3/1
  Divide3/1 -> V/1
  Integrator2/1 -> Add/2
  2/1 -> Divide2/2

== system System3/Battery1/Module3/SubModule_1/Cell9/2RC/RC2 ==
  Current : Inport
  R : Inport  Port=2
  C : Inport  Port=3
  2 : Constant
  Add : Sum
  Divide : Product  Inputs=*/
  Divide1 : Product  Inputs=*/
  Divide2 : Product  Inputs=/*
  Divide3 : Product  Inputs=**
  Integrator1 : Integrator
  Integrator2 : Integrator
  V : Outport
  wires:
  2/1 -> Divide2/2
  Integrator2/1 -> Add/2
  Divide3/1 -> V/1
  Current/1 -> Divide3/1
  Divide/1 -> Divide3/2
  Divide2/1 -> Integrator2/1
  R/1 -> Divide1/1, Add/1
  Add/1 -> Divide/2
  Divide1/1 -> Integrator1/1
  Integrator1/1 -> Divide/1
  C/1 -> Divide1/2, Divide2/1

== system System3/Battery1/Module3/SubModule_1/Cell9/2RC/Rint ==
  Current : Inport
  R : Inport  Port=2
  Divide3 : Product  Inputs=**
  V : Outport
  wires:
  R/1 -> Divide3/2
  Current/1 -> Divide3/1
  Divide3/1 -> V/1

== system System3/Battery1/Module3/SubModule_1/Cell9/SOCEstimator/SOCEstimator ==
  SOC_Initial : Inport
  Current : Inport  Port=2
  CellCapacity : Inport  Port=3
  Add1 : Sum  Inputs=+-
  Constant : Constant  Value=100  SampleTime=-1
  Constant1 : Constant  Value=3600  SampleTime=-1
  Delay : Delay  DelayLength=1  InitialConditionSource=Input port
      settings: InputPortMap=u0,p4
  Divide : Product  Inputs=*//
  Divide1 : Product  Inputs=*/
  Integrator : Integrator
  Saturation1 : Saturate  UpperLimit=1  LowerLimit=0
  SOC : Outport
  wires:
  Add1/1 -> Saturation1/1
  Constant/1 -> Divide1/2
  Divide1/1 -> Delay/2, Add1/1
  Divide/1 -> Add1/2
  Saturation1/1 -> Delay/1
  SOC_Initial/1 -> Divide1/1
  Current/1 -> Integrator/1
  Delay/1 -> SOC/1
  CellCapacity/1 -> Divide/2
  Constant1/1 -> Divide/3
  Integrator/1 -> Divide/1

== system System3/Battery1/Module3/SubModule_10/Cell1/2RC/RC1 ==
  Current : Inport
  R : Inport  Port=2
  C : Inport  Port=3
  2 : Constant
  Add : Sum
  Divide : Product  Inputs=*/
  Divide1 : Product  Inputs=*/
  Divide2 : Product  Inputs=/*
  Divide3 : Product  Inputs=**
  Integrator1 : Integrator
  Integrator2 : Integrator
  V : Outport
  wires:
  2/1 -> Divide2/2
  Integrator2/1 -> Add/2
  Divide3/1 -> V/1
  Current/1 -> Divide3/1
  Divide/1 -> Divide3/2
  Divide2/1 -> Integrator2/1
  R/1 -> Divide1/1, Add/1
  Add/1 -> Divide/2
  Divide1/1 -> Integrator1/1
  Integrator1/1 -> Divide/1
  C/1 -> Divide1/2, Divide2/1

== system System3/Battery1/Module3/SubModule_10/Cell1/2RC/RC2 ==
  Current : Inport
  R : Inport  Port=2
  C : Inport  Port=3
  2 : Constant
  Add : Sum
  Divide : Product  Inputs=*/
  Divide1 : Product  Inputs=*/
  Divide2 : Product  Inputs=/*
  Divide3 : Product  Inputs=**
  Integrator1 : Integrator
  Integrator2 : Integrator
  V : Outport
  wires:
  C/1 -> Divide2/1, Divide1/2
  Integrator1/1 -> Divide/1
  Divide1/1 -> Integrator1/1
  Add/1 -> Divide/2
  R/1 -> Add/1, Divide1/1
  Divide2/1 -> Integrator2/1
  Divide/1 -> Divide3/2
  Current/1 -> Divide3/1
  Divide3/1 -> V/1
  Integrator2/1 -> Add/2
  2/1 -> Divide2/2

== system System3/Battery1/Module3/SubModule_10/Cell1/2RC/Rint ==
  Current : Inport
  R : Inport  Port=2
  Divide3 : Product  Inputs=**
  V : Outport
  wires:
  Divide3/1 -> V/1
  Current/1 -> Divide3/1
  R/1 -> Divide3/2

== system System3/Battery1/Module3/SubModule_10/Cell1/SOCEstimator/SOCEstimator ==
  SOC_Initial : Inport
  Current : Inport  Port=2
  CellCapacity : Inport  Port=3
  Add1 : Sum  Inputs=+-
  Constant : Constant  Value=100  SampleTime=-1
  Constant1 : Constant  Value=3600  SampleTime=-1
  Delay : Delay  DelayLength=1  InitialConditionSource=Input port
      settings: InputPortMap=u0,p4
  Divide : Product  Inputs=*//
  Divide1 : Product  Inputs=*/
  Integrator : Integrator
  Saturation1 : Saturate  UpperLimit=1  LowerLimit=0
  SOC : Outport
  wires:
  Integrator/1 -> Divide/1
  Constant1/1 -> Divide/3
  CellCapacity/1 -> Divide/2
  Delay/1 -> SOC/1
  Current/1 -> Integrator/1
  SOC_Initial/1 -> Divide1/1
  Saturation1/1 -> Delay/1
  Divide/1 -> Add1/2
  Divide1/1 -> Add1/1, Delay/2
  Constant/1 -> Divide1/2
  Add1/1 -> Saturation1/1

== system System3/Battery1/Module3/SubModule_10/Cell10/2RC/RC1 ==
  Current : Inport
  R : Inport  Port=2
  C : Inport  Port=3
  2 : Constant
  Add : Sum
  Divide : Product  Inputs=*/
  Divide1 : Product  Inputs=*/
  Divide2 : Product  Inputs=/*
  Divide3 : Product  Inputs=**
  Integrator1 : Integrator
  Integrator2 : Integrator
  V : Outport
  wires:
  2/1 -> Divide2/2
  Integrator2/1 -> Add/2
  Divide3/1 -> V/1
  Current/1 -> Divide3/1
  Divide/1 -> Divide3/2
  Divide2/1 -> Integrator2/1
  R/1 -> Divide1/1, Add/1
  Add/1 -> Divide/2
  Divide1/1 -> Integrator1/1
  Integrator1/1 -> Divide/1
  C/1 -> Divide1/2, Divide2/1

== system System3/Battery1/Module3/SubModule_10/Cell10/2RC/RC2 ==
  Current : Inport
  R : Inport  Port=2
  C : Inport  Port=3
  2 : Constant
  Add : Sum
  Divide : Product  Inputs=*/
  Divide1 : Product  Inputs=*/
  Divide2 : Product  Inputs=/*
  Divide3 : Product  Inputs=**
  Integrator1 : Integrator
  Integrator2 : Integrator
  V : Outport
  wires:
  C/1 -> Divide2/1, Divide1/2
  Integrator1/1 -> Divide/1
  Divide1/1 -> Integrator1/1
  Add/1 -> Divide/2
  R/1 -> Add/1, Divide1/1
  Divide2/1 -> Integrator2/1
  Divide/1 -> Divide3/2
  Current/1 -> Divide3/1
  Divide3/1 -> V/1
  Integrator2/1 -> Add/2
  2/1 -> Divide2/2

== system System3/Battery1/Module3/SubModule_10/Cell10/2RC/Rint ==
  Current : Inport
  R : Inport  Port=2
  Divide3 : Product  Inputs=**
  V : Outport
  wires:
  Divide3/1 -> V/1
  Current/1 -> Divide3/1
  R/1 -> Divide3/2

== system System3/Battery1/Module3/SubModule_10/Cell10/SOCEstimator/SOCEstimator ==
  SOC_Initial : Inport
  Current : Inport  Port=2
  CellCapacity : Inport  Port=3
  Add1 : Sum  Inputs=+-
  Constant : Constant  Value=100  SampleTime=-1
  Constant1 : Constant  Value=3600  SampleTime=-1
  Delay : Delay  DelayLength=1  InitialConditionSource=Input port
      settings: InputPortMap=u0,p4
  Divide : Product  Inputs=*//
  Divide1 : Product  Inputs=*/
  Integrator : Integrator
  Saturation1 : Saturate  UpperLimit=1  LowerLimit=0
  SOC : Outport
  wires:
  Integrator/1 -> Divide/1
  Constant1/1 -> Divide/3
  CellCapacity/1 -> Divide/2
  Delay/1 -> SOC/1
  Current/1 -> Integrator/1
  SOC_Initial/1 -> Divide1/1
  Saturation1/1 -> Delay/1
  Divide/1 -> Add1/2
  Divide1/1 -> Add1/1, Delay/2
  Constant/1 -> Divide1/2
  Add1/1 -> Saturation1/1

== system System3/Battery1/Module3/SubModule_10/Cell11/2RC/RC1 ==
  Current : Inport
  R : Inport  Port=2
  C : Inport  Port=3
  2 : Constant
  Add : Sum
  Divide : Product  Inputs=*/
  Divide1 : Product  Inputs=*/
  Divide2 : Product  Inputs=/*
  Divide3 : Product  Inputs=**
  Integrator1 : Integrator
  Integrator2 : Integrator
  V : Outport
  wires:
  C/1 -> Divide2/1, Divide1/2
  Integrator1/1 -> Divide/1
  Divide1/1 -> Integrator1/1
  Add/1 -> Divide/2
  R/1 -> Add/1, Divide1/1
  Divide2/1 -> Integrator2/1
  Divide/1 -> Divide3/2
  Current/1 -> Divide3/1
  Divide3/1 -> V/1
  Integrator2/1 -> Add/2
  2/1 -> Divide2/2

== system System3/Battery1/Module3/SubModule_10/Cell11/2RC/RC2 ==
  Current : Inport
  R : Inport  Port=2
  C : Inport  Port=3
  2 : Constant
  Add : Sum
  Divide : Product  Inputs=*/
  Divide1 : Product  Inputs=*/
  Divide2 : Product  Inputs=/*
  Divide3 : Product  Inputs=**
  Integrator1 : Integrator
  Integrator2 : Integrator
  V : Outport
  wires:
  2/1 -> Divide2/2
  Integrator2/1 -> Add/2
  Divide3/1 -> V/1
  Current/1 -> Divide3/1
  Divide/1 -> Divide3/2
  Divide2/1 -> Integrator2/1
  R/1 -> Divide1/1, Add/1
  Add/1 -> Divide/2
  Divide1/1 -> Integrator1/1
  Integrator1/1 -> Divide/1
  C/1 -> Divide1/2, Divide2/1

== system System3/Battery1/Module3/SubModule_10/Cell11/2RC/Rint ==
  Current : Inport
  R : Inport  Port=2
  Divide3 : Product  Inputs=**
  V : Outport
  wires:
  R/1 -> Divide3/2
  Current/1 -> Divide3/1
  Divide3/1 -> V/1

== system System3/Battery1/Module3/SubModule_10/Cell11/SOCEstimator/SOCEstimator ==
  SOC_Initial : Inport
  Current : Inport  Port=2
  CellCapacity : Inport  Port=3
  Add1 : Sum  Inputs=+-
  Constant : Constant  Value=100  SampleTime=-1
  Constant1 : Constant  Value=3600  SampleTime=-1
  Delay : Delay  DelayLength=1  InitialConditionSource=Input port
      settings: InputPortMap=u0,p4
  Divide : Product  Inputs=*//
  Divide1 : Product  Inputs=*/
  Integrator : Integrator
  Saturation1 : Saturate  UpperLimit=1  LowerLimit=0
  SOC : Outport
  wires:
  Add1/1 -> Saturation1/1
  Constant/1 -> Divide1/2
  Divide1/1 -> Delay/2, Add1/1
  Divide/1 -> Add1/2
  Saturation1/1 -> Delay/1
  SOC_Initial/1 -> Divide1/1
  Current/1 -> Integrator/1
  Delay/1 -> SOC/1
  CellCapacity/1 -> Divide/2
  Constant1/1 -> Divide/3
  Integrator/1 -> Divide/1

== system System3/Battery1/Module3/SubModule_10/Cell12/2RC/RC1 ==
  Current : Inport
  R : Inport  Port=2
  C : Inport  Port=3
  2 : Constant
  Add : Sum
  Divide : Product  Inputs=*/
  Divide1 : Product  Inputs=*/
  Divide2 : Product  Inputs=/*
  Divide3 : Product  Inputs=**
  Integrator1 : Integrator
  Integrator2 : Integrator
  V : Outport
  wires:
  2/1 -> Divide2/2
  Integrator2/1 -> Add/2
  Divide3/1 -> V/1
  Current/1 -> Divide3/1
  Divide/1 -> Divide3/2
  Divide2/1 -> Integrator2/1
  R/1 -> Divide1/1, Add/1
  Add/1 -> Divide/2
  Divide1/1 -> Integrator1/1
  Integrator1/1 -> Divide/1
  C/1 -> Divide1/2, Divide2/1

== system System3/Battery1/Module3/SubModule_10/Cell12/2RC/RC2 ==
  Current : Inport
  R : Inport  Port=2
  C : Inport  Port=3
  2 : Constant
  Add : Sum
  Divide : Product  Inputs=*/
  Divide1 : Product  Inputs=*/
  Divide2 : Product  Inputs=/*
  Divide3 : Product  Inputs=**
  Integrator1 : Integrator
  Integrator2 : Integrator
  V : Outport
  wires:
  C/1 -> Divide2/1, Divide1/2
  Integrator1/1 -> Divide/1
  Divide1/1 -> Integrator1/1
  Add/1 -> Divide/2
  R/1 -> Add/1, Divide1/1
  Divide2/1 -> Integrator2/1
  Divide/1 -> Divide3/2
  Current/1 -> Divide3/1
  Divide3/1 -> V/1
  Integrator2/1 -> Add/2
  2/1 -> Divide2/2

== system System3/Battery1/Module3/SubModule_10/Cell12/2RC/Rint ==
  Current : Inport
  R : Inport  Port=2
  Divide3 : Product  Inputs=**
  V : Outport
  wires:
  Divide3/1 -> V/1
  Current/1 -> Divide3/1
  R/1 -> Divide3/2

== system System3/Battery1/Module3/SubModule_10/Cell12/SOCEstimator/SOCEstimator ==
  SOC_Initial : Inport
  Current : Inport  Port=2
  CellCapacity : Inport  Port=3
  Add1 : Sum  Inputs=+-
  Constant : Constant  Value=100  SampleTime=-1
  Constant1 : Constant  Value=3600  SampleTime=-1
  Delay : Delay  DelayLength=1  InitialConditionSource=Input port
      settings: InputPortMap=u0,p4
  Divide : Product  Inputs=*//
  Divide1 : Product  Inputs=*/
  Integrator : Integrator
  Saturation1 : Saturate  UpperLimit=1  LowerLimit=0
  SOC : Outport
  wires:
  Integrator/1 -> Divide/1
  Constant1/1 -> Divide/3
  CellCapacity/1 -> Divide/2
  Delay/1 -> SOC/1
  Current/1 -> Integrator/1
  SOC_Initial/1 -> Divide1/1
  Saturation1/1 -> Delay/1
  Divide/1 -> Add1/2
  Divide1/1 -> Add1/1, Delay/2
  Constant/1 -> Divide1/2
  Add1/1 -> Saturation1/1

== system System3/Battery1/Module3/SubModule_10/Cell13/2RC/RC1 ==
  Current : Inport
  R : Inport  Port=2
  C : Inport  Port=3
  2 : Constant
  Add : Sum
  Divide : Product  Inputs=*/
  Divide1 : Product  Inputs=*/
  Divide2 : Product  Inputs=/*
  Divide3 : Product  Inputs=**
  Integrator1 : Integrator
  Integrator2 : Integrator
  V : Outport
  wires:
  C/1 -> Divide2/1, Divide1/2
  Integrator1/1 -> Divide/1
  Divide1/1 -> Integrator1/1
  Add/1 -> Divide/2
  R/1 -> Add/1, Divide1/1
  Divide2/1 -> Integrator2/1
  Divide/1 -> Divide3/2
  Current/1 -> Divide3/1
  Divide3/1 -> V/1
  Integrator2/1 -> Add/2
  2/1 -> Divide2/2

== system System3/Battery1/Module3/SubModule_10/Cell13/2RC/RC2 ==
  Current : Inport
  R : Inport  Port=2
  C : Inport  Port=3
  2 : Constant
  Add : Sum
  Divide : Product  Inputs=*/
  Divide1 : Product  Inputs=*/
  Divide2 : Product  Inputs=/*
  Divide3 : Product  Inputs=**
  Integrator1 : Integrator
  Integrator2 : Integrator
  V : Outport
  wires:
  2/1 -> Divide2/2
  Integrator2/1 -> Add/2
  Divide3/1 -> V/1
  Current/1 -> Divide3/1
  Divide/1 -> Divide3/2
  Divide2/1 -> Integrator2/1
  R/1 -> Divide1/1, Add/1
  Add/1 -> Divide/2
  Divide1/1 -> Integrator1/1
  Integrator1/1 -> Divide/1
  C/1 -> Divide1/2, Divide2/1

== system System3/Battery1/Module3/SubModule_10/Cell13/2RC/Rint ==
  Current : Inport
  R : Inport  Port=2
  Divide3 : Product  Inputs=**
  V : Outport
  wires:
  R/1 -> Divide3/2
  Current/1 -> Divide3/1
  Divide3/1 -> V/1

== system System3/Battery1/Module3/SubModule_10/Cell13/SOCEstimator/SOCEstimator ==
  SOC_Initial : Inport
  Current : Inport  Port=2
  CellCapacity : Inport  Port=3
  Add1 : Sum  Inputs=+-
  Constant : Constant  Value=100  SampleTime=-1
  Constant1 : Constant  Value=3600  SampleTime=-1
  Delay : Delay  DelayLength=1  InitialConditionSource=Input port
      settings: InputPortMap=u0,p4
  Divide : Product  Inputs=*//
  Divide1 : Product  Inputs=*/
  Integrator : Integrator
  Saturation1 : Saturate  UpperLimit=1  LowerLimit=0
  SOC : Outport
  wires:
  Add1/1 -> Saturation1/1
  Constant/1 -> Divide1/2
  Divide1/1 -> Delay/2, Add1/1
  Divide/1 -> Add1/2
  Saturation1/1 -> Delay/1
  SOC_Initial/1 -> Divide1/1
  Current/1 -> Integrator/1
  Delay/1 -> SOC/1
  CellCapacity/1 -> Divide/2
  Constant1/1 -> Divide/3
  Integrator/1 -> Divide/1
